simulink model "sampleModel1676"  (R2023a)
settings: Solver=VariableStepAuto  StartTime=0.0  StopTime=10.0  RelTol=1e-3
libraries: hdlsllib x4, simulink x1
settings Model: Creator=user1  LastModifiedBy=user1

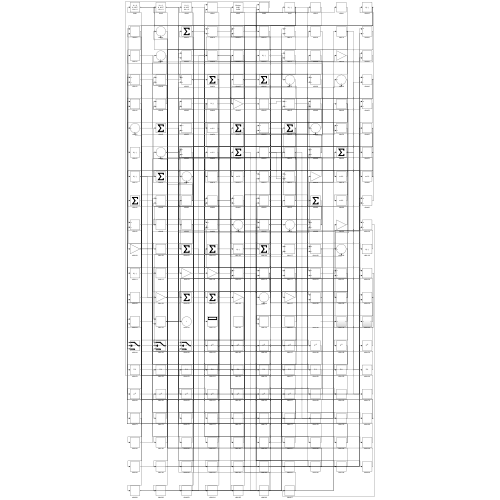
[thumbnail: Simulink's stored preview of the top-level diagram]
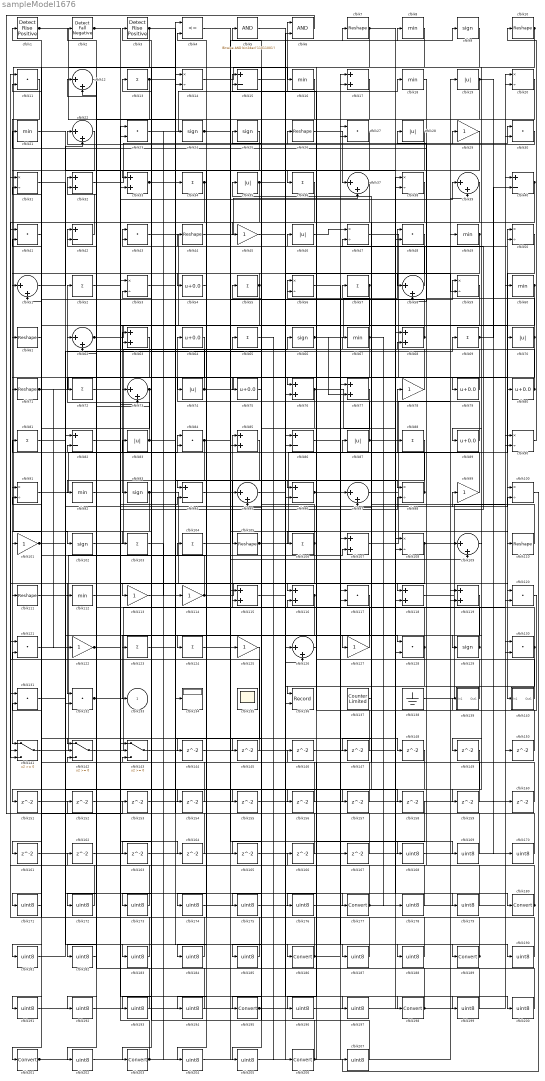
== system sampleModel1676 ==
  cfblk1 : hdlsllib/Logic and Bit Operations/Detect Rise Positive  vinit=0  OutDataTypeStr=boolean
  cfblk{7,10,26,44,61,71,105,110..111} (9 alike) : Reshape
  cfblk{14,20,31,38,47,50,53,56,59,90..91,98,100,108} (14 alike) : Product  Inputs=*/  RndMeth=Zero  SaturateOnIntegerOverflow=on
  cfblk{29,45,78,99,101,113..114,122,125,127} (10 alike) : Gain
  cfblk{9,24..25,66,93,102,129} (7 alike) : Signum
  cfblk{13,34,36,52,55,57,65,69,72,81,88,103..104,106,123..124} (16 alike) : Sum  Inputs=+
  cfblk{17,32..33,63,68,76..77,85,107,115..116,118..119} (13 alike) : Sum
  cfblk{12,22,37,39,51,58,62,73,95,97,109,126} (12 alike) : Sum  Inputs=|++
  cfblk{11,23,27,30,41,43,48,84,117,120..121,128,130..132} (15 alike) : DotProduct  OutDataTypeStr=Inherit: Inherit via internal rule
  cfblk{8,16,18,21,49,60,67,92,112} (9 alike) : MinMax
  cfblk134 : Display
  cfblk135 : Scope
      settings: Floating=on
  cfblk136 : Record  FileSettingsInternal="{\"entries\":[{\"content\":{\"excelSettings\":{\"content\":{},\"type\":\"Streamout.ExcelSettings\"}},\"type\":\"Streamout.FileSettingStorage\",\"uuid\":\"\"}],\"packageUris\":[\"http:\\/\\/schema.mathworks.com\\/mf0\\/streamout_blocks\\/R2020a\"],\"version\":\"1.0\"}"  Layout=[1 1]  SignalsInternal="{\"entries\":[{\"content\":{\"signals\":[{\"content\":{\"blockPath\":[],\"dimensions\":[1],\"domain\":\"\",\"lineColor\":\"#a2142f\",\"plots\":[1],\"port\":1,\"sid\":[\"\"],\"signalID\":2796,\"signalName\":\"cfblk40\"},\"type\":\"RecordBlkView.Signal\",\"uuid\":\"\"},{\"content\":{\"blockPath\":[],\"dimensions\":[1],\"domain\":\"\",\"lineColor\":\"#139fff\",\"plots\":[1],\"port\":2,\"sid\":[\"\"],\"signalID\":2800,\"signalName\":\"cfblk130\"},\"type\":\"RecordBlkView.Signal\",\"uuid\":\"\"}]},\"type\":\"RecordBlkView.InputSignals\",\"uuid\":\"\"}],\"packageUris\":[\"http:\\/\\/schema.mathworks.com\\/mf0\\/streamout_blocks\\/R2020a\"],\"version\":\"1.0\"}"  VisualizationBindings="{\"xyplotplugin\":{\"info\":[{\"series\":[{\"bindingParametersList\":[{\"parameter\":\"X-Axis\",\"signalID\":2796,\"signalName\":\"cfblk40\"},{\"parameter\":\"Y-Axis\",\"signalID\":2800,\"signalName\":\"cfblk130\"}],\"seriesID\":31174}],\"subplotID\":1}]}}"  CompatibilityTag=XY  st=-1
  cfblk137 : hdlsllib/Sources/Counter Limited  uplimit=7  tsamp=-1
  cfblk138 : Ground
  cfblk139 : Subsystem
      settings: LibrarySourceBlock=|
      | hdlsllib/Ports &
      | Subsystems/Subsystem
  cfblk140 : Subsystem
      settings: LibrarySourceBlock=|
      | hdlsllib/Ports &
      | Subsystems/Subsystem
  cfblk141 : Switch  SaturateOnIntegerOverflow=off  InputSameDT=off
  cfblk142 : Switch  SaturateOnIntegerOverflow=off  InputSameDT=off
  cfblk143 : Switch  SaturateOnIntegerOverflow=off  InputSameDT=off
  cfblk{144..167} (24 alike) : Delay  SampleTime=1
  cfblk{15,40,42,82,86,94,96} (7 alike) : Sum  Inputs=+-
  cfblk{168..176,178..179,181..185,187..188,190..194,196..197,199..200,202,204..205,207} (31 alike) : DataTypeConversion  OutDataTypeStr=uint8  SaturateOnIntegerOverflow=off  RndMeth=Floor
  cfblk{177,180,186,189,195,198,201,203,206} (9 alike) : DataTypeConversion  SaturateOnIntegerOverflow=off  RndMeth=Floor
  cfblk{19,28,35,46,70,74,83,87} (8 alike) : Abs  SaturateOnIntegerOverflow=off
  cfblk2 : hdlsllib/Logic and Bit Operations/Detect Fall Negative  vinit=0  OutDataTypeStr=boolean
  cfblk3 : hdlsllib/Logic and Bit Operations/Detect Rise Positive  vinit=0  OutDataTypeStr=boolean
  cfblk4 : RelationalOperator  Operator=<=  OutDataTypeStr=boolean  InputSameDT=off
  cfblk5 : simulink/Logic and Bit Operations/Bitwise Operator  logicop=AND  UseBitMask=on  BitMask=bin2dec('11011001')  BitMaskRealWorld=Stored Integer
      settings: LibrarySourceBlock=|
      | hdlsllib/Logic and Bit
      | Operations/Bitwise
      | Operator
  cfblk{54,64,75,79..80,89} (6 alike) : Bias  Bias=0.0  SaturateOnIntegerOverflow=off
  cfblk6 : Logic  AllPortsSameDT=off  OutDataTypeStr=boolean
  cfblk133 : Outport  VectorParamsAs1DForOutWhenUnconnected=off
  wires:
  cfblk103/1 -> cfblk114/1
  cfblk71/1 -> cfblk79/1, cfblk122/1, cfblk128/1
  cfblk84/1 -> cfblk9/1, cfblk59/1, cfblk202/1
  cfblk3/1 -> cfblk102/1, cfblk187/1
  cfblk102/1 -> cfblk66/1
  cfblk62/1 -> cfblk89/1, cfblk70/1
  cfblk63/1 -> cfblk141/1
  cfblk101/1 -> cfblk99/1, cfblk158/1
  cfblk17/1 -> cfblk203/1
  cfblk46/1 -> cfblk47/1
  cfblk99/1 -> cfblk78/1
  cfblk121/1 -> cfblk177/1
  cfblk123/1 -> cfblk34/1
  cfblk67/1 -> cfblk57/1, cfblk94/1, cfblk173/1, cfblk178/1
  cfblk138/1 -> cfblk47/2
  cfblk114/1 -> cfblk116/1, cfblk51/2
  cfblk57/1 -> cfblk93/1, cfblk56/2
  cfblk30/1 -> cfblk22/1
  cfblk126/1 -> cfblk46/1
  cfblk66/1 -> cfblk48/1, cfblk77/2, cfblk188/1
  cfblk75/1 -> cfblk25/1
  cfblk125/1 -> cfblk201/1
  cfblk129/1 -> cfblk127/1, cfblk83/1
  cfblk53/1 -> cfblk186/1
  cfblk29/1 -> cfblk36/1
  cfblk11/1 -> cfblk91/1
  cfblk23/1 -> cfblk6/1
  cfblk32/1 -> cfblk30/1
  cfblk83/1 -> cfblk52/1, cfblk29/1, cfblk62/2
  cfblk50/1 -> cfblk140/1(In1)
  cfblk105/1 -> cfblk50/1, cfblk126/2
  cfblk19/1 -> cfblk72/1, cfblk159/1, cfblk160/1
  cfblk38/1 -> cfblk113/1
  cfblk86/1 -> cfblk189/1
  cfblk90/1 -> cfblk10/1
  cfblk51/1 -> cfblk22/2
  cfblk22/1 -> cfblk61/1
  cfblk141/1 -> cfblk6/2
  cfblk96/1 -> cfblk117/2, cfblk50/2
  cfblk47/1 -> cfblk100/1
  cfblk106/1 -> cfblk62/1, cfblk141/3
  cfblk89/1 -> cfblk64/1
  cfblk107/1 -> cfblk19/1
  cfblk130/1 -> cfblk87/1, cfblk136/2
  cfblk26/1 -> cfblk37/1
  cfblk142/1 -> cfblk60/1
  cfblk91/1 -> cfblk84/1
  cfblk116/1 -> cfblk144/1, cfblk184/1
  cfblk111/1 -> cfblk132/1
  cfblk18/1 -> cfblk58/1
  cfblk98/1 -> cfblk42/1, cfblk81/1
  cfblk80/1 -> cfblk5/1, cfblk75/1
  cfblk113/1 -> cfblk100/2
  cfblk55/1 -> cfblk51/1, cfblk73/1, cfblk161/1
  cfblk35/1 -> cfblk7/1, cfblk59/2, cfblk194/1
  cfblk139/1(Out1) -> cfblk63/1
  cfblk132/1 -> cfblk85/1, cfblk73/2, cfblk94/2, cfblk164/1
  cfblk94/1 -> cfblk105/1
  cfblk137/1 -> cfblk67/1
  cfblk14/1 -> cfblk16/1
  cfblk45/1 -> cfblk18/1
  cfblk64/1 -> cfblk71/1
  cfblk131/1 -> cfblk69/1
  cfblk13/1 -> cfblk92/1, cfblk148/1
  cfblk68/1 -> cfblk11/2, cfblk15/2
  cfblk21/1 -> cfblk33/1
  cfblk128/1 -> cfblk95/2, cfblk156/1
  cfblk43/1 -> cfblk107/1
  cfblk24/1 -> cfblk110/1, cfblk109/2
  cfblk58/1 -> cfblk3/1
  cfblk87/1 -> cfblk38/1, cfblk56/1
  cfblk108/1 -> cfblk90/1, cfblk193/1
  cfblk42/1 -> cfblk32/1
  cfblk49/1 -> cfblk76/1, cfblk124/1
  cfblk110/1 -> cfblk35/1
  cfblk40/1 -> cfblk136/1, cfblk58/2
  cfblk10/1 -> cfblk129/1, cfblk128/2, cfblk196/1
  cfblk79/1 -> cfblk63/2
  cfblk140/1(Out1) -> cfblk15/1
  cfblk65/1 -> cfblk206/1
  cfblk44/1 -> cfblk37/2
  cfblk56/1 -> cfblk97/1
  cfblk82/1 -> cfblk180/1
  cfblk5/1 -> cfblk126/1
  cfblk37/1 -> cfblk106/1
  cfblk69/1 -> cfblk40/2, cfblk170/1
  cfblk118/1 -> cfblk30/2
  cfblk93/1 -> cfblk120/1, cfblk132/2
  cfblk76/1 -> cfblk108/2, cfblk95/1
  cfblk97/1 -> cfblk49/1
  cfblk73/1 -> cfblk101/1, cfblk43/1
  cfblk9/1 -> cfblk45/1
  cfblk112/1 -> cfblk107/2
  cfblk115/1 -> cfblk198/1
  cfblk78/1 -> cfblk44/1
  cfblk54/1 -> cfblk74/1
  cfblk120/1 -> cfblk139/1(In1)
  cfblk143/1 -> cfblk88/1
  cfblk117/1 -> cfblk133/1
  cfblk7/1 -> cfblk23/2, cfblk123/1, cfblk111/1, cfblk179/1
  cfblk36/1 -> cfblk112/1
  cfblk60/1 -> cfblk103/1, cfblk85/2
  cfblk1/1 -> cfblk134/1, cfblk14/2
  cfblk15/1 -> cfblk8/1
  cfblk20/1 -> cfblk195/1
  cfblk28/1 -> cfblk96/1
  cfblk92/1 -> cfblk39/1
  cfblk70/1 -> cfblk21/1, cfblk157/1
  cfblk34/1 -> cfblk141/2, cfblk54/1
  cfblk74/1 -> cfblk32/2, cfblk80/1
  cfblk127/1 -> cfblk42/2
  cfblk27/1 -> cfblk142/1
  cfblk2/1 -> cfblk118/1, cfblk38/2
  cfblk122/1 -> cfblk33/2, cfblk98/2
  cfblk33/1 -> cfblk118/2, cfblk98/1
  cfblk124/1 -> cfblk26/1
  cfblk144/1 -> cfblk68/1
  cfblk8/1 -> cfblk145/1
  cfblk145/1 -> cfblk11/1
  cfblk146/1 -> cfblk27/2
  cfblk39/1 -> cfblk147/1
  cfblk147/1 -> cfblk116/2
  cfblk109/1 -> cfblk149/1
  cfblk150/1 -> cfblk77/1
  cfblk61/1 -> cfblk151/1
  cfblk151/1 -> cfblk76/2
  cfblk152/1 -> cfblk90/2
  cfblk6/1 -> cfblk153/1
  cfblk153/1 -> cfblk108/1
  cfblk25/1 -> cfblk154/1
  cfblk154/1 -> cfblk14/1
  cfblk81/1 -> cfblk155/1
  cfblk156/1 -> cfblk91/2
  cfblk157/1 -> cfblk84/2
  cfblk159/1 -> cfblk97/2
  cfblk160/1 -> cfblk142/2
  cfblk161/1 -> cfblk143/1
  cfblk162/1 -> cfblk130/2
  cfblk85/1 -> cfblk163/1
  cfblk163/1 -> cfblk40/1
  cfblk164/1 -> cfblk142/3
  cfblk59/1 -> cfblk165/1
  cfblk166/1 -> cfblk1/1
  cfblk167/1 -> cfblk131/2
  cfblk4/1 -> cfblk168/1
  cfblk168/1 -> cfblk28/1
  cfblk104/1 -> cfblk169/1
  cfblk169/1 -> cfblk4/1
  cfblk170/1 -> cfblk4/2
  cfblk41/1 -> cfblk171/1
  cfblk48/1 -> cfblk172/1
  cfblk172/1 -> cfblk41/1
  cfblk173/1 -> cfblk41/2
  cfblk119/1 -> cfblk174/1
  cfblk174/1 -> cfblk130/1
  cfblk77/1 -> cfblk175/1
  cfblk175/1 -> cfblk119/1
  cfblk158/1 -> cfblk176/1
  cfblk176/1 -> cfblk119/2
  cfblk177/1 -> cfblk162/1, cfblk2/1, cfblk55/1
  cfblk178/1 -> cfblk121/1
  cfblk179/1 -> cfblk121/2
  cfblk180/1 -> cfblk43/2, cfblk68/2
  cfblk149/1 -> cfblk181/1
  cfblk181/1 -> cfblk82/1
  cfblk16/1 -> cfblk182/1
  cfblk182/1 -> cfblk82/2
  cfblk31/1 -> cfblk183/1
  cfblk183/1 -> cfblk131/1
  cfblk184/1 -> cfblk31/1
  cfblk148/1 -> cfblk185/1
  cfblk185/1 -> cfblk31/2
  cfblk186/1 -> cfblk167/1, cfblk166/1, cfblk143/2
  cfblk187/1 -> cfblk53/1
  cfblk188/1 -> cfblk53/2
  cfblk189/1 -> cfblk104/1, cfblk117/1
  cfblk72/1 -> cfblk190/1
  cfblk190/1 -> cfblk86/1
  cfblk171/1 -> cfblk191/1
  cfblk191/1 -> cfblk86/2
  cfblk12/1 -> cfblk192/1
  cfblk192/1 -> cfblk120/2
  cfblk193/1 -> cfblk12/1
  cfblk194/1 -> cfblk12/2
  cfblk195/1 -> cfblk150/1, cfblk48/2
  cfblk196/1 -> cfblk20/1
  cfblk95/1 -> cfblk197/1
  cfblk197/1 -> cfblk20/2
  cfblk198/1 -> cfblk152/1, cfblk143/3
  cfblk165/1 -> cfblk199/1
  cfblk199/1 -> cfblk115/1
  cfblk52/1 -> cfblk200/1
  cfblk200/1 -> cfblk115/2
  cfblk201/1 -> cfblk96/2, cfblk27/1
  cfblk202/1 -> cfblk125/1
  cfblk203/1 -> cfblk39/2, cfblk24/1, cfblk23/1
  cfblk88/1 -> cfblk204/1
  cfblk204/1 -> cfblk17/1
  cfblk155/1 -> cfblk205/1
  cfblk205/1 -> cfblk17/2
  cfblk206/1 -> cfblk146/1, cfblk109/1, cfblk13/1
  cfblk100/1 -> cfblk207/1
  cfblk207/1 -> cfblk65/1

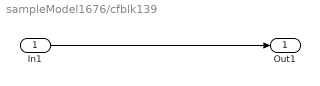
== system sampleModel1676/cfblk139 ==
  In1 : Inport
  Out1 : Outport
  wires:
  In1/1 -> Out1/1

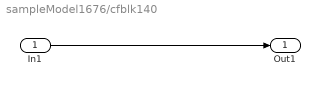
== system sampleModel1676/cfblk140 ==
  In1 : Inport
  Out1 : Outport
  wires:
  In1/1 -> Out1/1
